simulink model "IEEE_39_IBR_Simplified"  (R2023b)
settings: Solver=FixedStepAuto  StartTime=0  StopTime=20  FixedStep=Ts  MaxStep=1/60  RelTol=1e-3  AbsTol=1e-2  EnableMultiTasking=on
PreLoadFcn:
  | NE39bus_data;
  | PSSMODEL=1;
  | LPSS=0;
  | WAPSS=0;
  | WAPSS2=0;
values from neighbouring files (symbols this model uses):
  Dt = 0    [SG_para.m]
  dw0_sm = 0    [SG_para.m]
  Emax = 1    [SG_para.m]
  Emin = 0.5    [SG_para.m]
  Fg = [0.1,0.1,0.1]    [SG_para.m]
  fn_sm = 60*ones(1,10)    [SG_para.m]
  H_sm = [5,3.03,3.58,2.86,2.6,3.48,2.64,2.43,3.45,4.2]*10    [SG_para.m]
  ia0_sm = 0.75*0    (= 0)    [SG_para.m]
  ib0_sm = 0.75*0    (= 0)    [SG_para.m]
  ic0_sm = 0.75*0    (= 0)    [SG_para.m]
  Kd_sm = 6*ones(1,10)    [SG_para.m]
  Ke = 200    [SG_para.m]
  Kg = [0.95,0.95,0.95]    [SG_para.m]
  Ks = 2    [SG_para.m]
  line = [     1	2	0.0035	0.0411	0.6987	0	100	345 ... (first row only)    [SG_para.m]
  p = 1    [SG_para.m]
  pha0_sm = -24.95*0    (= 0)    [SG_para.m]
  phb0_sm = -144.94*0    (= 0)    [SG_para.m]
  phc0_sm = 95.05*0    (= 0)    [SG_para.m]
  Pn_sm = [1000,1000,1000,1000,1000,1000,1000,1000,1000,1000]    [SG_para.m]
  Pref_sm = [1000 520.81 650 632 508 650 560 540 830 250]./Pn_sm    [SG_para.m]
  R = 1e-3    (= 0.001)    [SG_para.m]
  Rg = [0.05,0.05,0.05]    [SG_para.m]
  rs = 2.8544e-3    (= 0.0028544)    [SG_para.m]
  s = 1    [SG_para.m]
  s1 = 10    [SG_para.m]
  T1 = 0.05    [SG_para.m]
  T2 = 0.5    [SG_para.m]
  T3 = 0.5    [SG_para.m]
  Te = 0.05    [SG_para.m]
  Tfa = 3    [SG_para.m]
  Tfb = 10    [SG_para.m]
  Tg = [10,10,10]    [SG_para.m]
  theta0_sm = -94.3*0    (= 0)    [SG_para.m]
  Ts = 5e-5    (= 5e-05)    [SG_para.m]
  Ts1 = 0.18    [SG_para.m]
  Ts2 = 2    [SG_para.m]
  Ts3 = 5    [SG_para.m]
  Ts4 = 10    [SG_para.m]
  Ts5 = 15    [SG_para.m]
  Un_sm = [345,22,22,22,22,22,22,22,345,22]    [SG_para.m]
  Vmax = inf    [SG_para.m]
  Vmin = 0    [SG_para.m]
  Vref_sm = 1*ones(1,10)    [SG_para.m]
  xd = xd_t    (= 0.296)    [SG_para.m]
undefined symbols (not defined in the file or in its folder): D1, D11, Delta, Ka, Kf, Ta, Tf
libraries: spsThreePhaseVIMeasurementLib x41, spsThreePhaseFaultLib x39, spsThreePhaseSeriesRLCBranchLib x36, spsThreePhaseParallelRLCLoadLib x20, spsThreePhaseTransformerTwoWindingsLib x13, spsSimplifiedSynchronousMachinepuUnitsLib x10, spsLoadFlowBusLib x10, Inverter_based_Resources_IBRs x10, spsThreePhaseBreakerLib x2, spsSequenceAnalyzerLib x2, spsMultimeterLib x1, eePowerMeasurement x1
(part 4 of 5)

== system IEEE_39_IBR_Simplified/A2/G1 ==
  Controllers : Subsystem
  Simplified Synchronous Machine pu Units : spsSimplifiedSynchronousMachinepuUnitsLib/Simplified Synchronous Machine pu Units  ConnectionType=3-wire Y  MechanicalLoad=Mechanical power Pm  MeasurementBus=off  NominalParameters="[ Pn_sm(1)*1e6  Un_sm(1)*1e3  fn_sm(1) ]"  Mechanical=[ H_sm(1) Kd_sm(1) p]  InternalRL="[rs  xd]"  InitialConditions=[dw0_sm theta0_sm ia0_sm ib0_sm ic0_sm pha0_sm phb0_sm phc0_sm]  IterativeDiscreteModel=Trapezoidal non iterative  TsBlock=-1  TsPowergui=0  LoadFlowParameters=[1 0 0 0 0]  Units=0  BusType=swing  Pref=0  Qref=0  Qmin=-inf  Qmax=+inf  PLF=0  QLF=0
      settings: LibrarySourceBlock=|
      | sps_lib/Electrical Machines/Simplified Synchronous
      | Machine pu Units
  A : PMIOPort  Side=Left
  B : PMIOPort  Port=2  Side=Left
  C : PMIOPort  Port=3  Side=Left
  wires:
  Controllers/1(Pm) -> Simplified Synchronous Machine pu Units/1
  Simplified Synchronous Machine pu Units/1 -> Controllers/1(m)
  Controllers/2(Vref) -> Simplified Synchronous Machine pu Units/2
  connections:
  A/RConn1 -- Simplified Synchronous Machine pu Units/RConn1
  B/RConn1 -- Simplified Synchronous Machine pu Units/RConn2
  C/RConn1 -- Simplified Synchronous Machine pu Units/RConn3

== system IEEE_39_IBR_Simplified/A2/G2 ==
  Controllers : Subsystem
  Simplified Synchronous Machine pu Units : spsSimplifiedSynchronousMachinepuUnitsLib/Simplified Synchronous Machine pu Units  ConnectionType=3-wire Y  MechanicalLoad=Mechanical power Pm  MeasurementBus=off  NominalParameters="[ Pn_sm(2)*1e6  Un_sm(2)*1e3  fn_sm(2) ]"  Mechanical=[ H_sm(2) Kd_sm(2) p]  InternalRL="[rs  xd]"  InitialConditions=[dw0_sm theta0_sm ia0_sm ib0_sm ic0_sm pha0_sm phb0_sm phc0_sm]  IterativeDiscreteModel=Trapezoidal non iterative  TsBlock=-1  TsPowergui=0  LoadFlowParameters=[1,0,0,0,0]  Units=0  BusType=PV  Pref=0  Qref=0  Qmin=-inf  Qmax=+inf  PLF=0  QLF=0
      settings: LibrarySourceBlock=|
      | sps_lib/Electrical Machines/Simplified Synchronous
      | Machine pu Units
  A : PMIOPort  Side=Left
  B : PMIOPort  Port=2  Side=Left
  C : PMIOPort  Port=3  Side=Left
  wires:
  Controllers/1(Pm) -> Simplified Synchronous Machine pu Units/1
  Simplified Synchronous Machine pu Units/1 -> Controllers/1(m)
  Controllers/2(Vref) -> Simplified Synchronous Machine pu Units/2
  connections:
  Simplified Synchronous Machine pu Units/RConn2 -- B/RConn1
  Simplified Synchronous Machine pu Units/RConn3 -- C/RConn1
  Simplified Synchronous Machine pu Units/RConn1 -- A/RConn1

== system IEEE_39_IBR_Simplified/A2/G3 ==
  Controllers : Subsystem
  Simplified Synchronous Machine pu Units : spsSimplifiedSynchronousMachinepuUnitsLib/Simplified Synchronous Machine pu Units  ConnectionType=3-wire Y  MechanicalLoad=Mechanical power Pm  MeasurementBus=off  NominalParameters="[ Pn_sm(3)*1e6  Un_sm(3)*1e3  fn_sm(3) ]"  Mechanical=[ H_sm(3) Kd_sm(3) p]  InternalRL="[rs  xd]"  InitialConditions=[dw0_sm theta0_sm ia0_sm ib0_sm ic0_sm pha0_sm phb0_sm phc0_sm]  IterativeDiscreteModel=Trapezoidal non iterative  TsBlock=-1  TsPowergui=0  LoadFlowParameters=[1,0,0,0,0]  Units=0  BusType=PV  Pref=0  Qref=0  Qmin=-inf  Qmax=+inf  PLF=0  QLF=0
      settings: LibrarySourceBlock=|
      | sps_lib/Electrical Machines/Simplified Synchronous
      | Machine pu Units
  A : PMIOPort  Side=Left
  B : PMIOPort  Port=2  Side=Left
  C : PMIOPort  Port=3  Side=Left
  wires:
  Controllers/1(Pm) -> Simplified Synchronous Machine pu Units/1
  Simplified Synchronous Machine pu Units/1 -> Controllers/1(m)
  Controllers/2(Vref) -> Simplified Synchronous Machine pu Units/2
  connections:
  Simplified Synchronous Machine pu Units/RConn2 -- B/RConn1
  Simplified Synchronous Machine pu Units/RConn3 -- C/RConn1
  Simplified Synchronous Machine pu Units/RConn1 -- A/RConn1

== system IEEE_39_IBR_Simplified/A3/G4 ==
  Controllers : Subsystem
  Simplified Synchronous Machine pu Units : spsSimplifiedSynchronousMachinepuUnitsLib/Simplified Synchronous Machine pu Units  ConnectionType=3-wire Y  MechanicalLoad=Mechanical power Pm  MeasurementBus=off  NominalParameters="[ Pn_sm(4)*1e6  Un_sm(4)*1e3  fn_sm(4) ]"  Mechanical=[ H_sm(4) Kd_sm(4) p]  InternalRL="[rs  xd]"  InitialConditions=[dw0_sm theta0_sm ia0_sm ib0_sm ic0_sm pha0_sm phb0_sm phc0_sm]  IterativeDiscreteModel=Trapezoidal non iterative  TsBlock=-1  TsPowergui=0  LoadFlowParameters=[1,0,0,0,0]  Units=0  BusType=PV  Pref=0  Qref=0  Qmin=-inf  Qmax=+inf  PLF=0  QLF=0
      settings: LibrarySourceBlock=|
      | sps_lib/Electrical Machines/Simplified Synchronous
      | Machine pu Units
  A : PMIOPort  Side=Left
  B : PMIOPort  Port=2  Side=Left
  C : PMIOPort  Port=3  Side=Left
  wires:
  Controllers/1(Pm) -> Simplified Synchronous Machine pu Units/1
  Simplified Synchronous Machine pu Units/1 -> Controllers/1(m)
  Controllers/2(Vref) -> Simplified Synchronous Machine pu Units/2
  connections:
  Simplified Synchronous Machine pu Units/RConn2 -- B/RConn1
  Simplified Synchronous Machine pu Units/RConn3 -- C/RConn1
  Simplified Synchronous Machine pu Units/RConn1 -- A/RConn1

== system IEEE_39_IBR_Simplified/A3/G5 ==
  Controllers : Subsystem
  Simplified Synchronous Machine pu Units : spsSimplifiedSynchronousMachinepuUnitsLib/Simplified Synchronous Machine pu Units  ConnectionType=3-wire Y  MechanicalLoad=Mechanical power Pm  MeasurementBus=off  NominalParameters="[ Pn_sm(5)*1e6  Un_sm(5)*1e3  fn_sm(5) ]"  Mechanical=[ H_sm(5) Kd_sm(5) p]  InternalRL="[rs  xd]"  InitialConditions=[dw0_sm theta0_sm ia0_sm ib0_sm ic0_sm pha0_sm phb0_sm phc0_sm]  IterativeDiscreteModel=Trapezoidal non iterative  TsBlock=-1  TsPowergui=0  LoadFlowParameters=[1,0,0,0,0]  Units=0  BusType=PV  Pref=0  Qref=0  Qmin=-inf  Qmax=+inf  PLF=0  QLF=0
      settings: LibrarySourceBlock=|
      | sps_lib/Electrical Machines/Simplified Synchronous
      | Machine pu Units
  A : PMIOPort  Side=Left
  B : PMIOPort  Port=2  Side=Left
  C : PMIOPort  Port=3  Side=Left
  wires:
  Controllers/1(Pm) -> Simplified Synchronous Machine pu Units/1
  Simplified Synchronous Machine pu Units/1 -> Controllers/1(m)
  Controllers/2(Vref) -> Simplified Synchronous Machine pu Units/2
  connections:
  Simplified Synchronous Machine pu Units/RConn2 -- B/RConn1
  Simplified Synchronous Machine pu Units/RConn3 -- C/RConn1
  Simplified Synchronous Machine pu Units/RConn1 -- A/RConn1

== system IEEE_39_IBR_Simplified/A3/G6 ==
  Controllers : Subsystem
  Simplified Synchronous Machine pu Units : spsSimplifiedSynchronousMachinepuUnitsLib/Simplified Synchronous Machine pu Units  ConnectionType=3-wire Y  MechanicalLoad=Mechanical power Pm  MeasurementBus=off  NominalParameters="[ Pn_sm(6)*1e6  Un_sm(6)*1e3  fn_sm(6) ]"  Mechanical=[ H_sm(6) Kd_sm(6) p]  InternalRL="[rs  xd]"  InitialConditions=[dw0_sm theta0_sm ia0_sm ib0_sm ic0_sm pha0_sm phb0_sm phc0_sm]  IterativeDiscreteModel=Trapezoidal non iterative  TsBlock=-1  TsPowergui=0  LoadFlowParameters=[1,0,0,0,0]  Units=0  BusType=PV  Pref=0  Qref=0  Qmin=-inf  Qmax=+inf  PLF=0  QLF=0
      settings: LibrarySourceBlock=|
      | sps_lib/Electrical Machines/Simplified Synchronous
      | Machine pu Units
  A : PMIOPort  Side=Left
  B : PMIOPort  Port=2  Side=Left
  C : PMIOPort  Port=3  Side=Left
  wires:
  Controllers/1(Pm) -> Simplified Synchronous Machine pu Units/1
  Simplified Synchronous Machine pu Units/1 -> Controllers/1(m)
  Controllers/2(Vref) -> Simplified Synchronous Machine pu Units/2
  connections:
  Simplified Synchronous Machine pu Units/RConn2 -- B/RConn1
  Simplified Synchronous Machine pu Units/RConn3 -- C/RConn1
  Simplified Synchronous Machine pu Units/RConn1 -- A/RConn1

== system IEEE_39_IBR_Simplified/A3/G7 ==
  Controllers : Subsystem
  Simplified Synchronous Machine pu Units : spsSimplifiedSynchronousMachinepuUnitsLib/Simplified Synchronous Machine pu Units  ConnectionType=3-wire Y  MechanicalLoad=Mechanical power Pm  MeasurementBus=off  NominalParameters="[ Pn_sm(7)*1e6  Un_sm(7)*1e3  fn_sm(7) ]"  Mechanical=[ H_sm(7) Kd_sm(7) p]  InternalRL="[rs  xd]"  InitialConditions=[dw0_sm theta0_sm ia0_sm ib0_sm ic0_sm pha0_sm phb0_sm phc0_sm]  IterativeDiscreteModel=Trapezoidal non iterative  TsBlock=-1  TsPowergui=0  LoadFlowParameters=[1,0,0,0,0]  Units=0  BusType=PV  Pref=0  Qref=0  Qmin=-inf  Qmax=+inf  PLF=0  QLF=0
      settings: LibrarySourceBlock=|
      | sps_lib/Electrical Machines/Simplified Synchronous
      | Machine pu Units
  A : PMIOPort  Side=Left
  B : PMIOPort  Port=2  Side=Left
  C : PMIOPort  Port=3  Side=Left
  wires:
  Controllers/1(Pm) -> Simplified Synchronous Machine pu Units/1
  Simplified Synchronous Machine pu Units/1 -> Controllers/1(m)
  Controllers/2(Vref) -> Simplified Synchronous Machine pu Units/2
  connections:
  Simplified Synchronous Machine pu Units/RConn2 -- B/RConn1
  Simplified Synchronous Machine pu Units/RConn3 -- C/RConn1
  Simplified Synchronous Machine pu Units/RConn1 -- A/RConn1

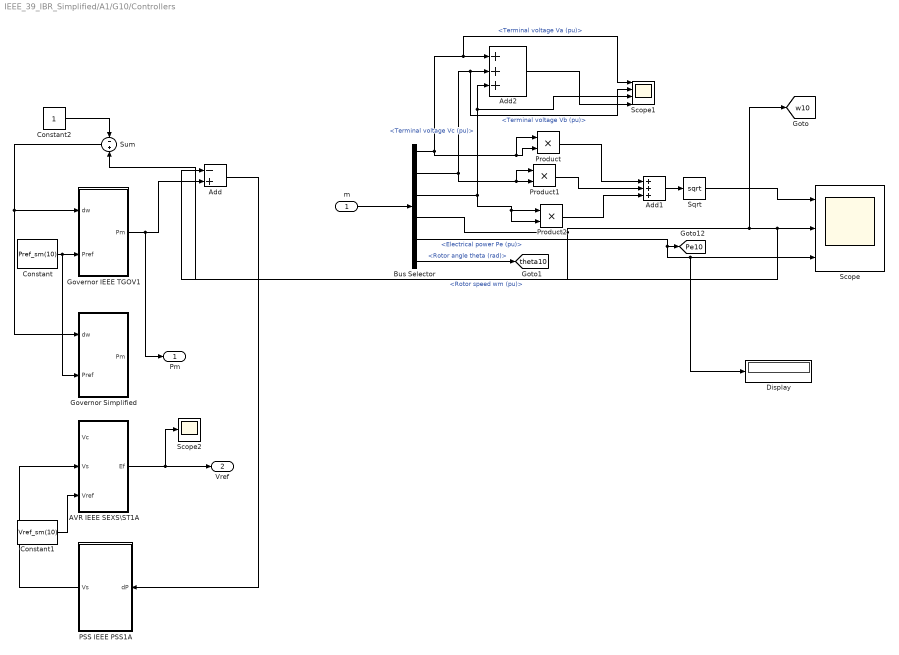
== system IEEE_39_IBR_Simplified/A1/G10/Controllers ==
  m : Inport
  AVR IEEE SEXS\ST1A : Subsystem
  Add : Sum  Inputs=-+
  Add1 : Sum  Inputs=+++
  Add2 : Sum  Inputs=+++
  Bus Selector : BusSelector  OutputSignals=Terminal voltage Va (pu),Terminal voltage Vb (pu),Terminal voltage Vc (pu),Rotor speed wm (pu),Electrical power Pe (pu),Rotor angle theta (rad)
  Constant : Constant  Value=Pref_sm(10)
  Constant1 : Constant  Value=Vref_sm(10)
  Constant2 : Constant
  Display : Display
  Governor Simplified : Subsystem
  Governor IEEE TGOV1 : Subsystem
  PSS IEEE PSS1A : Subsystem
  Product : Product
  Product1 : Product
  Product2 : Product
  Scope : Scope  NumInputPorts=3
  Scope1 : Scope  NumInputPorts=4
  Scope2 : Scope
  Sqrt : Sqrt
  Sum : Sum  Inputs=-+
  Pm : Outport  VectorParamsAs1DForOutWhenUnconnected=off
  Vref : Outport  Port=2  VectorParamsAs1DForOutWhenUnconnected=off
  tag scope: Pe10=global, theta10=global, w10=global
  wires:
  Governor IEEE TGOV1/1(Pm) -> Pm/1, Add/2
  Constant/1 -> Governor Simplified/2(Pref), Governor IEEE TGOV1/2(Pref)
  Add/1 -> PSS IEEE PSS1A/1(dP)
  Constant1/1 -> AVR IEEE SEXS\ST1A/3(Vref)
  PSS IEEE PSS1A/1(Vs) -> AVR IEEE SEXS\ST1A/2(Vs)
  m/1 -> Bus Selector/1
  Bus Selector/4 -> [w10], Sum/2, Scope/2, Add/1  "<Rotor speed wm (pu)>"
  Bus Selector/2 -> Product1/1, Product1/2, Scope1/2, Add2/2  "<Terminal voltage Vb (pu)>"
  Bus Selector/3 -> Product2/1, Product2/2, Scope1/3, Add2/3  "<Terminal voltage Vc (pu)>"
  Bus Selector/1 -> Product/1, Product/2, Scope1/1, Add2/1  "<Terminal voltage Va (pu)>"
  Bus Selector/5 -> Display/1, Scope/3, [Pe10]  "<Electrical power Pe (pu)>"
  Add1/1 -> Sqrt/1
  Product/1 -> Add1/1
  Product1/1 -> Add1/2
  Product2/1 -> Add1/3
  Constant2/1 -> Sum/1
  Sum/1 -> Governor IEEE TGOV1/1(dw), Governor Simplified/1(dw)
  Sqrt/1 -> Scope/1
  Add2/1 -> Scope1/4
  Bus Selector/6 -> [theta10]  "<Rotor angle theta (rad)>"
  AVR IEEE SEXS\ST1A/1(Ef) -> Scope2/1, Vref/1

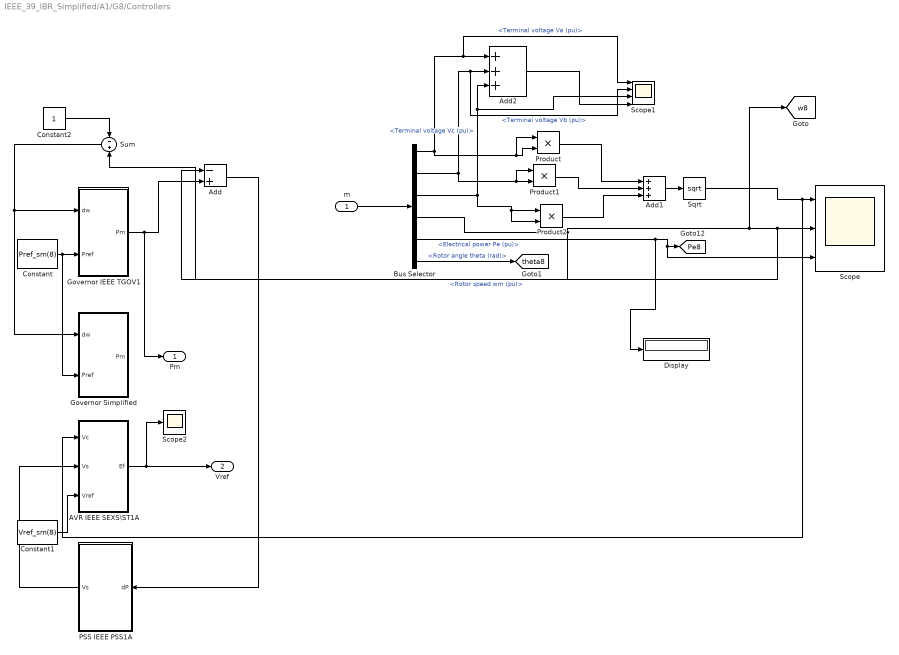
== system IEEE_39_IBR_Simplified/A1/G8/Controllers ==
  m : Inport
  AVR IEEE SEXS\ST1A : Subsystem
  Add : Sum  Inputs=-+
  Add1 : Sum  Inputs=+++
  Add2 : Sum  Inputs=+++
  Bus Selector : BusSelector  OutputSignals=Terminal voltage Va (pu),Terminal voltage Vb (pu),Terminal voltage Vc (pu),Rotor speed wm (pu),Electrical power Pe (pu),Rotor angle theta (rad)
  Constant : Constant  Value=Pref_sm(8)
  Constant1 : Constant  Value=Vref_sm(8)
  Constant2 : Constant
  Display : Display
  Governor Simplified : Subsystem
  Governor IEEE TGOV1 : Subsystem
  PSS IEEE PSS1A : Subsystem
  Product : Product
  Product1 : Product
  Product2 : Product
  Scope : Scope  NumInputPorts=3
  Scope1 : Scope  NumInputPorts=4
  Scope2 : Scope
  Sqrt : Sqrt
  Sum : Sum  Inputs=-+
  Pm : Outport  VectorParamsAs1DForOutWhenUnconnected=off
  Vref : Outport  Port=2  VectorParamsAs1DForOutWhenUnconnected=off
  tag scope: Pe8=global, theta8=global, w8=global
  wires:
  Governor IEEE TGOV1/1(Pm) -> Pm/1, Add/2
  Constant/1 -> Governor Simplified/2(Pref), Governor IEEE TGOV1/2(Pref)
  Add/1 -> PSS IEEE PSS1A/1(dP)
  Constant1/1 -> AVR IEEE SEXS\ST1A/3(Vref)
  PSS IEEE PSS1A/1(Vs) -> AVR IEEE SEXS\ST1A/2(Vs)
  m/1 -> Bus Selector/1
  Bus Selector/4 -> [w8], Sum/2, Scope/2, Add/1  "<Rotor speed wm (pu)>"
  Bus Selector/2 -> Product1/1, Product1/2, Scope1/2, Add2/2  "<Terminal voltage Vb (pu)>"
  Bus Selector/3 -> Product2/1, Product2/2, Scope1/3, Add2/3  "<Terminal voltage Vc (pu)>"
  Bus Selector/1 -> Product/1, Product/2, Scope1/1, Add2/1  "<Terminal voltage Va (pu)>"
  Bus Selector/5 -> Display/1, Scope/3, [Pe8]  "<Electrical power Pe (pu)>"
  Add1/1 -> Sqrt/1
  Product/1 -> Add1/1
  Product1/1 -> Add1/2
  Product2/1 -> Add1/3
  Constant2/1 -> Sum/1
  Sum/1 -> Governor IEEE TGOV1/1(dw), Governor Simplified/1(dw)
  Sqrt/1 -> AVR IEEE SEXS\ST1A/1(Vc), Scope/1
  Add2/1 -> Scope1/4
  Bus Selector/6 -> [theta8]  "<Rotor angle theta (rad)>"
  AVR IEEE SEXS\ST1A/1(Ef) -> Scope2/1, Vref/1

== system IEEE_39_IBR_Simplified/A1/G9/Controllers ==
  m : Inport
  AVR IEEE SEXS\ST1A : Subsystem
  Add : Sum  Inputs=-+
  Add1 : Sum  Inputs=+++
  Add2 : Sum  Inputs=+++
  Bus Selector : BusSelector  OutputSignals=Terminal voltage Va (pu),Terminal voltage Vb (pu),Terminal voltage Vc (pu),Rotor speed wm (pu),Electrical power Pe (pu),Rotor angle theta (rad)
  Constant : Constant  Value=Pref_sm(9)
  Constant1 : Constant  Value=Vref_sm(9)
  Constant2 : Constant
  Display : Display
  Governor Simplified : Subsystem
  Governor IEEE TGOV1 : Subsystem
  PSS IEEE PSS1A : Subsystem
  Product : Product
  Product1 : Product
  Product2 : Product
  Scope : Scope  NumInputPorts=3
  Scope1 : Scope  NumInputPorts=4
  Sqrt : Sqrt
  Sum : Sum  Inputs=-+
  Pm : Outport  VectorParamsAs1DForOutWhenUnconnected=off
  Vref : Outport  Port=2  VectorParamsAs1DForOutWhenUnconnected=off
  tag scope: Pe9=global, theta9=global, w9=global
  wires:
  Governor IEEE TGOV1/1(Pm) -> Pm/1, Add/2
  Constant/1 -> Governor Simplified/2(Pref), Governor IEEE TGOV1/2(Pref)
  Add/1 -> PSS IEEE PSS1A/1(dP)
  Constant1/1 -> AVR IEEE SEXS\ST1A/3(Vref)
  PSS IEEE PSS1A/1(Vs) -> AVR IEEE SEXS\ST1A/2(Vs)
  m/1 -> Bus Selector/1
  Bus Selector/4 -> [w9], Sum/2, Scope/2, Add/1  "<Rotor speed wm (pu)>"
  Bus Selector/2 -> Product1/1, Product1/2, Scope1/2, Add2/2  "<Terminal voltage Vb (pu)>"
  Bus Selector/3 -> Product2/1, Product2/2, Scope1/3, Add2/3  "<Terminal voltage Vc (pu)>"
  Bus Selector/1 -> Product/1, Product/2, Scope1/1, Add2/1  "<Terminal voltage Va (pu)>"
  Bus Selector/5 -> Display/1, Scope/3, [Pe9]  "<Electrical power Pe (pu)>"
  Add1/1 -> Sqrt/1
  Product/1 -> Add1/1
  Product1/1 -> Add1/2
  Product2/1 -> Add1/3
  Constant2/1 -> Sum/1
  Sum/1 -> Governor IEEE TGOV1/1(dw), Governor Simplified/1(dw)
  Sqrt/1 -> Scope/1
  Add2/1 -> Scope1/4
  Bus Selector/6 -> [theta9]  "<Rotor angle theta (rad)>"
  AVR IEEE SEXS\ST1A/1(Ef) -> Vref/1

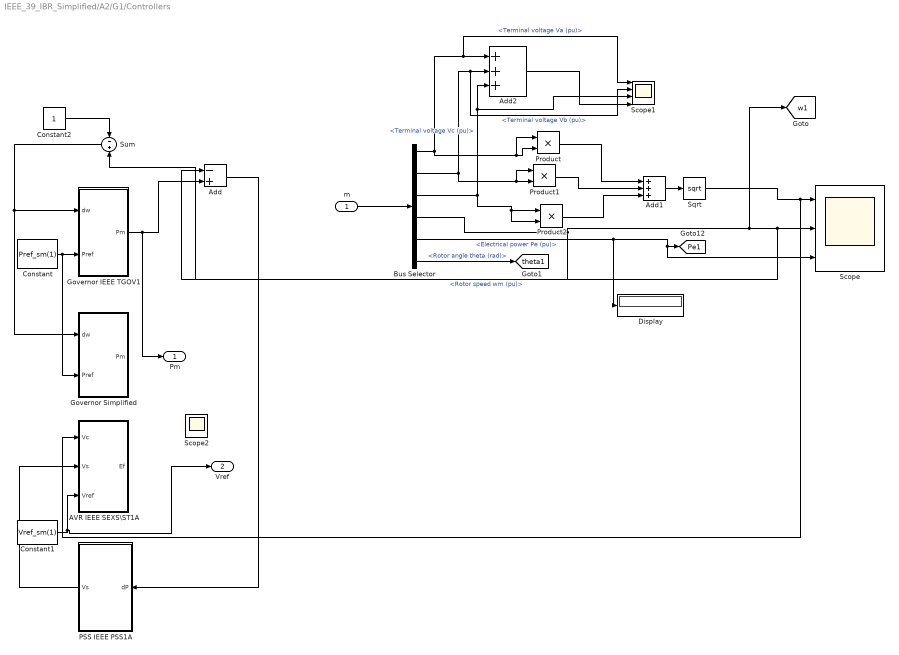
== system IEEE_39_IBR_Simplified/A2/G1/Controllers ==
  m : Inport
  AVR IEEE SEXS\ST1A : Subsystem
  Add : Sum  Inputs=-+
  Add1 : Sum  Inputs=+++
  Add2 : Sum  Inputs=+++
  Bus Selector : BusSelector  OutputSignals=Terminal voltage Va (pu),Terminal voltage Vb (pu),Terminal voltage Vc (pu),Rotor speed wm (pu),Electrical power Pe (pu),Rotor angle theta (rad)
  Constant : Constant  Value=Pref_sm(1)
  Constant1 : Constant  Value=Vref_sm(1)
  Constant2 : Constant
  Display : Display
  Governor Simplified : Subsystem
  Governor IEEE TGOV1 : Subsystem
  PSS IEEE PSS1A : Subsystem
  Product : Product
  Product1 : Product
  Product2 : Product
  Scope : Scope  NumInputPorts=3
  Scope1 : Scope  NumInputPorts=4
  Scope2 : Scope
  Sqrt : Sqrt
  Sum : Sum  Inputs=-+
  Pm : Outport  VectorParamsAs1DForOutWhenUnconnected=off
  Vref : Outport  Port=2  VectorParamsAs1DForOutWhenUnconnected=off
  tag scope: Pe1=global, theta1=global, w1=global
  wires:
  Governor IEEE TGOV1/1(Pm) -> Pm/1, Add/2
  Constant/1 -> Governor Simplified/2(Pref), Governor IEEE TGOV1/2(Pref)
  Add/1 -> PSS IEEE PSS1A/1(dP)
  Constant1/1 -> Vref/1, AVR IEEE SEXS\ST1A/3(Vref)
  PSS IEEE PSS1A/1(Vs) -> AVR IEEE SEXS\ST1A/2(Vs)
  m/1 -> Bus Selector/1
  Bus Selector/4 -> [w1], Sum/2, Scope/2, Add/1  "<Rotor speed wm (pu)>"
  Bus Selector/2 -> Product1/1, Product1/2, Scope1/2, Add2/2  "<Terminal voltage Vb (pu)>"
  Bus Selector/3 -> Product2/1, Product2/2, Scope1/3, Add2/3  "<Terminal voltage Vc (pu)>"
  Bus Selector/1 -> Product/1, Product/2, Scope1/1, Add2/1  "<Terminal voltage Va (pu)>"
  Bus Selector/5 -> Display/1, Scope/3, [Pe1]  "<Electrical power Pe (pu)>"
  Add1/1 -> Sqrt/1
  Product/1 -> Add1/1
  Product1/1 -> Add1/2
  Product2/1 -> Add1/3
  Constant2/1 -> Sum/1
  Sum/1 -> Governor IEEE TGOV1/1(dw), Governor Simplified/1(dw)
  Sqrt/1 -> AVR IEEE SEXS\ST1A/1(Vc), Scope/1
  Add2/1 -> Scope1/4
  Bus Selector/6 -> [theta1]  "<Rotor angle theta (rad)>"

== system IEEE_39_IBR_Simplified/A2/G2/Controllers ==
  m : Inport
  AVR IEEE SEXS\ST1A : Subsystem
  Add : Sum  Inputs=-+
  Add1 : Sum  Inputs=+++
  Add2 : Sum  Inputs=+++
  Bus Selector : BusSelector  OutputSignals=Terminal voltage Va (pu),Terminal voltage Vb (pu),Terminal voltage Vc (pu),Rotor speed wm (pu),Electrical power Pe (pu),Rotor angle theta (rad)
  Constant : Constant  Value=Pref_sm(2)
  Constant1 : Constant  Value=Vref_sm(2)
  Constant2 : Constant
  Display : Display
  Governor Simplified : Subsystem
  Governor IEEE TGOV1 : Subsystem
  PSS IEEE PSS1A : Subsystem
  Product : Product
  Product1 : Product
  Product2 : Product
  Scope : Scope  NumInputPorts=3
  Scope1 : Scope  NumInputPorts=4
  Sqrt : Sqrt
  Sum : Sum  Inputs=-+
  Pm : Outport  VectorParamsAs1DForOutWhenUnconnected=off
  Vref : Outport  Port=2  VectorParamsAs1DForOutWhenUnconnected=off
  tag scope: Pe2=global, theta2=global, w2=global
  wires:
  Governor IEEE TGOV1/1(Pm) -> Pm/1, Add/2
  Constant/1 -> Governor Simplified/2(Pref), Governor IEEE TGOV1/2(Pref)
  Add/1 -> PSS IEEE PSS1A/1(dP)
  Constant1/1 -> AVR IEEE SEXS\ST1A/3(Vref)
  PSS IEEE PSS1A/1(Vs) -> AVR IEEE SEXS\ST1A/2(Vs)
  m/1 -> Bus Selector/1
  Bus Selector/4 -> [w2], Sum/2, Scope/2, Add/1  "<Rotor speed wm (pu)>"
  Bus Selector/2 -> Product1/1, Product1/2, Scope1/2, Add2/2  "<Terminal voltage Vb (pu)>"
  Bus Selector/3 -> Product2/1, Product2/2, Scope1/3, Add2/3  "<Terminal voltage Vc (pu)>"
  Bus Selector/1 -> Product/1, Product/2, Scope1/1, Add2/1  "<Terminal voltage Va (pu)>"
  Bus Selector/5 -> Display/1, Scope/3, [Pe2]  "<Electrical power Pe (pu)>"
  Add1/1 -> Sqrt/1
  Product/1 -> Add1/1
  Product1/1 -> Add1/2
  Product2/1 -> Add1/3
  Constant2/1 -> Sum/1
  Sum/1 -> Governor IEEE TGOV1/1(dw), Governor Simplified/1(dw)
  Sqrt/1 -> Scope/1
  Add2/1 -> Scope1/4
  Bus Selector/6 -> [theta2]  "<Rotor angle theta (rad)>"
  AVR IEEE SEXS\ST1A/1(Ef) -> Vref/1

== system IEEE_39_IBR_Simplified/A2/G3/Controllers ==
  m : Inport
  AVR IEEE SEXS\ST1A : Subsystem
  Add : Sum  Inputs=-+
  Add1 : Sum  Inputs=+++
  Add2 : Sum  Inputs=+++
  Bus Selector : BusSelector  OutputSignals=Terminal voltage Va (pu),Terminal voltage Vb (pu),Terminal voltage Vc (pu),Rotor speed wm (pu),Electrical power Pe (pu),Rotor angle theta (rad)
  Constant : Constant  Value=Pref_sm(3)
  Constant1 : Constant  Value=Vref_sm(3)
  Constant2 : Constant
  Display : Display
  Governor Simplified : Subsystem
  Governor IEEE TGOV1 : Subsystem
  PSS IEEE PSS1A : Subsystem
  Product : Product
  Product1 : Product
  Product2 : Product
  Scope : Scope  NumInputPorts=3
  Scope1 : Scope  NumInputPorts=4
  Sqrt : Sqrt
  Sum : Sum  Inputs=-+
  Pm : Outport  VectorParamsAs1DForOutWhenUnconnected=off
  Vref : Outport  Port=2  VectorParamsAs1DForOutWhenUnconnected=off
  tag scope: Pe3=global, theta3=global, w3=global
  wires:
  Governor IEEE TGOV1/1(Pm) -> Pm/1, Add/2
  Constant/1 -> Governor Simplified/2(Pref), Governor IEEE TGOV1/2(Pref)
  Add/1 -> PSS IEEE PSS1A/1(dP)
  Constant1/1 -> AVR IEEE SEXS\ST1A/3(Vref)
  PSS IEEE PSS1A/1(Vs) -> AVR IEEE SEXS\ST1A/2(Vs)
  m/1 -> Bus Selector/1
  Bus Selector/4 -> [w3], Sum/2, Scope/2, Add/1  "<Rotor speed wm (pu)>"
  Bus Selector/2 -> Product1/1, Product1/2, Scope1/2, Add2/2  "<Terminal voltage Vb (pu)>"
  Bus Selector/3 -> Product2/1, Product2/2, Scope1/3, Add2/3  "<Terminal voltage Vc (pu)>"
  Bus Selector/1 -> Product/1, Product/2, Scope1/1, Add2/1  "<Terminal voltage Va (pu)>"
  Bus Selector/5 -> Display/1, Scope/3, [Pe3]  "<Electrical power Pe (pu)>"
  Add1/1 -> Sqrt/1
  Product/1 -> Add1/1
  Product1/1 -> Add1/2
  Product2/1 -> Add1/3
  Constant2/1 -> Sum/1
  Sum/1 -> Governor IEEE TGOV1/1(dw), Governor Simplified/1(dw)
  Sqrt/1 -> Scope/1
  Add2/1 -> Scope1/4
  Bus Selector/6 -> [theta3]  "<Rotor angle theta (rad)>"
  AVR IEEE SEXS\ST1A/1(Ef) -> Vref/1

== system IEEE_39_IBR_Simplified/A3/G4/Controllers ==
  m : Inport
  AVR IEEE SEXS\ST1A : Subsystem
  Add : Sum  Inputs=-+
  Add1 : Sum  Inputs=+++
  Add2 : Sum  Inputs=+++
  Bus Selector : BusSelector  OutputSignals=Terminal voltage Va (pu),Terminal voltage Vb (pu),Terminal voltage Vc (pu),Rotor speed wm (pu),Electrical power Pe (pu),Rotor angle theta (rad)
  Constant : Constant  Value=Pref_sm(4)
  Constant1 : Constant  Value=Vref_sm(4)
  Constant2 : Constant
  Display : Display
  Governor Simplified : Subsystem
  Governor IEEE TGOV1 : Subsystem
  PSS IEEE PSS1A : Subsystem
  Product : Product
  Product1 : Product
  Product2 : Product
  Scope : Scope  NumInputPorts=3
  Scope1 : Scope  NumInputPorts=4
  Sqrt : Sqrt
  Sum : Sum  Inputs=-+
  Pm : Outport  VectorParamsAs1DForOutWhenUnconnected=off
  Vref : Outport  Port=2  VectorParamsAs1DForOutWhenUnconnected=off
  tag scope: Pe4=global, theta4=global, w4=global
  wires:
  Governor IEEE TGOV1/1(Pm) -> Pm/1, Add/2
  Constant/1 -> Governor Simplified/2(Pref), Governor IEEE TGOV1/2(Pref)
  Add/1 -> PSS IEEE PSS1A/1(dP)
  Constant1/1 -> AVR IEEE SEXS\ST1A/3(Vref)
  PSS IEEE PSS1A/1(Vs) -> AVR IEEE SEXS\ST1A/2(Vs)
  m/1 -> Bus Selector/1
  Bus Selector/4 -> [w4], Sum/2, Scope/2, Add/1  "<Rotor speed wm (pu)>"
  Bus Selector/2 -> Product1/1, Product1/2, Scope1/2, Add2/2  "<Terminal voltage Vb (pu)>"
  Bus Selector/3 -> Product2/1, Product2/2, Scope1/3, Add2/3  "<Terminal voltage Vc (pu)>"
  Bus Selector/1 -> Product/1, Product/2, Scope1/1, Add2/1  "<Terminal voltage Va (pu)>"
  Bus Selector/5 -> Display/1, Scope/3, [Pe4]  "<Electrical power Pe (pu)>"
  Add1/1 -> Sqrt/1
  Product/1 -> Add1/1
  Product1/1 -> Add1/2
  Product2/1 -> Add1/3
  Constant2/1 -> Sum/1
  Sum/1 -> Governor IEEE TGOV1/1(dw), Governor Simplified/1(dw)
  Sqrt/1 -> Scope/1
  Add2/1 -> Scope1/4
  Bus Selector/6 -> [theta4]  "<Rotor angle theta (rad)>"
  AVR IEEE SEXS\ST1A/1(Ef) -> Vref/1

== system IEEE_39_IBR_Simplified/A3/G5/Controllers ==
  m : Inport
  AVR IEEE SEXS\ST1A : Subsystem
  Add : Sum  Inputs=-+
  Add1 : Sum  Inputs=+++
  Add2 : Sum  Inputs=+++
  Bus Selector : BusSelector  OutputSignals=Terminal voltage Va (pu),Terminal voltage Vb (pu),Terminal voltage Vc (pu),Rotor speed wm (pu),Electrical power Pe (pu),Rotor angle theta (rad)
  Constant : Constant  Value=Pref_sm(5)
  Constant1 : Constant  Value=Vref_sm(5)
  Constant2 : Constant
  Display : Display
  Governor Simplified : Subsystem
  Governor IEEE TGOV1 : Subsystem
  PSS IEEE PSS1A : Subsystem
  Product : Product
  Product1 : Product
  Product2 : Product
  Scope : Scope  NumInputPorts=3
  Scope1 : Scope  NumInputPorts=4
  Sqrt : Sqrt
  Sum : Sum  Inputs=-+
  Pm : Outport  VectorParamsAs1DForOutWhenUnconnected=off
  Vref : Outport  Port=2  VectorParamsAs1DForOutWhenUnconnected=off
  tag scope: Pe5=global, theta5=global, w5=global
  wires:
  Governor IEEE TGOV1/1(Pm) -> Pm/1, Add/2
  Constant/1 -> Governor Simplified/2(Pref), Governor IEEE TGOV1/2(Pref)
  Add/1 -> PSS IEEE PSS1A/1(dP)
  Constant1/1 -> AVR IEEE SEXS\ST1A/3(Vref)
  PSS IEEE PSS1A/1(Vs) -> AVR IEEE SEXS\ST1A/2(Vs)
  m/1 -> Bus Selector/1
  Bus Selector/4 -> [w5], Sum/2, Scope/2, Add/1  "<Rotor speed wm (pu)>"
  Bus Selector/2 -> Product1/1, Product1/2, Scope1/2, Add2/2  "<Terminal voltage Vb (pu)>"
  Bus Selector/3 -> Product2/1, Product2/2, Scope1/3, Add2/3  "<Terminal voltage Vc (pu)>"
  Bus Selector/1 -> Product/1, Product/2, Scope1/1, Add2/1  "<Terminal voltage Va (pu)>"
  Bus Selector/5 -> Display/1, Scope/3, [Pe5]  "<Electrical power Pe (pu)>"
  Add1/1 -> Sqrt/1
  Product/1 -> Add1/1
  Product1/1 -> Add1/2
  Product2/1 -> Add1/3
  Constant2/1 -> Sum/1
  Sum/1 -> Governor IEEE TGOV1/1(dw), Governor Simplified/1(dw)
  Sqrt/1 -> Scope/1
  Add2/1 -> Scope1/4
  Bus Selector/6 -> [theta5]  "<Rotor angle theta (rad)>"
  AVR IEEE SEXS\ST1A/1(Ef) -> Vref/1

== system IEEE_39_IBR_Simplified/A3/G6/Controllers ==
  m : Inport
  AVR IEEE SEXS\ST1A : Subsystem
  Add : Sum  Inputs=-+
  Add1 : Sum  Inputs=+++
  Add2 : Sum  Inputs=+++
  Bus Selector : BusSelector  OutputSignals=Terminal voltage Va (pu),Terminal voltage Vb (pu),Terminal voltage Vc (pu),Rotor speed wm (pu),Electrical power Pe (pu),Rotor angle theta (rad)
  Constant : Constant  Value=Pref_sm(6)
  Constant1 : Constant  Value=Vref_sm(6)
  Constant2 : Constant
  Display : Display
  Governor Simplified : Subsystem
  Governor IEEE TGOV1 : Subsystem
  PSS IEEE PSS1A : Subsystem
  Product : Product
  Product1 : Product
  Product2 : Product
  Scope : Scope  NumInputPorts=3
  Scope1 : Scope  NumInputPorts=4
  Sqrt : Sqrt
  Sum : Sum  Inputs=-+
  Pm : Outport  VectorParamsAs1DForOutWhenUnconnected=off
  Vref : Outport  Port=2  VectorParamsAs1DForOutWhenUnconnected=off
  tag scope: Pe6=global, theta6=global, w6=global
  wires:
  Governor IEEE TGOV1/1(Pm) -> Pm/1, Add/2
  Constant/1 -> Governor Simplified/2(Pref), Governor IEEE TGOV1/2(Pref)
  Add/1 -> PSS IEEE PSS1A/1(dP)
  Constant1/1 -> AVR IEEE SEXS\ST1A/3(Vref)
  PSS IEEE PSS1A/1(Vs) -> AVR IEEE SEXS\ST1A/2(Vs)
  m/1 -> Bus Selector/1
  Bus Selector/4 -> [w6], Sum/2, Scope/2, Add/1  "<Rotor speed wm (pu)>"
  Bus Selector/2 -> Product1/1, Product1/2, Scope1/2, Add2/2  "<Terminal voltage Vb (pu)>"
  Bus Selector/3 -> Product2/1, Product2/2, Scope1/3, Add2/3  "<Terminal voltage Vc (pu)>"
  Bus Selector/1 -> Product/1, Product/2, Scope1/1, Add2/1  "<Terminal voltage Va (pu)>"
  Bus Selector/5 -> Display/1, Scope/3, [Pe6]  "<Electrical power Pe (pu)>"
  Add1/1 -> Sqrt/1
  Product/1 -> Add1/1
  Product1/1 -> Add1/2
  Product2/1 -> Add1/3
  Constant2/1 -> Sum/1
  Sum/1 -> Governor IEEE TGOV1/1(dw), Governor Simplified/1(dw)
  Sqrt/1 -> Scope/1
  Add2/1 -> Scope1/4
  Bus Selector/6 -> [theta6]  "<Rotor angle theta (rad)>"
  AVR IEEE SEXS\ST1A/1(Ef) -> Vref/1

== system IEEE_39_IBR_Simplified/A3/G7/Controllers ==
  m : Inport
  AVR IEEE SEXS\ST1A : Subsystem
  Add : Sum  Inputs=-+
  Add1 : Sum  Inputs=+++
  Add2 : Sum  Inputs=+++
  Bus Selector : BusSelector  OutputSignals=Terminal voltage Va (pu),Terminal voltage Vb (pu),Terminal voltage Vc (pu),Rotor speed wm (pu),Electrical power Pe (pu),Rotor angle theta (rad)
  Constant : Constant  Value=Pref_sm(7)
  Constant1 : Constant  Value=Vref_sm(7)
  Constant2 : Constant
  Display : Display
  Governor Simplified : Subsystem
  Governor IEEE TGOV1 : Subsystem
  PSS IEEE PSS1A : Subsystem
  Product : Product
  Product1 : Product
  Product2 : Product
  Scope : Scope  NumInputPorts=3
  Scope1 : Scope  NumInputPorts=4
  Sqrt : Sqrt
  Sum : Sum  Inputs=-+
  Pm : Outport  VectorParamsAs1DForOutWhenUnconnected=off
  Vref : Outport  Port=2  VectorParamsAs1DForOutWhenUnconnected=off
  tag scope: Pe7=global, theta7=global, w7=global
  wires:
  Governor IEEE TGOV1/1(Pm) -> Pm/1, Add/2
  Constant/1 -> Governor Simplified/2(Pref), Governor IEEE TGOV1/2(Pref)
  Add/1 -> PSS IEEE PSS1A/1(dP)
  Constant1/1 -> AVR IEEE SEXS\ST1A/3(Vref)
  PSS IEEE PSS1A/1(Vs) -> AVR IEEE SEXS\ST1A/2(Vs)
  m/1 -> Bus Selector/1
  Bus Selector/4 -> [w7], Sum/2, Scope/2, Add/1  "<Rotor speed wm (pu)>"
  Bus Selector/2 -> Product1/1, Product1/2, Scope1/2, Add2/2  "<Terminal voltage Vb (pu)>"
  Bus Selector/3 -> Product2/1, Product2/2, Scope1/3, Add2/3  "<Terminal voltage Vc (pu)>"
  Bus Selector/1 -> Product/1, Product/2, Scope1/1, Add2/1  "<Terminal voltage Va (pu)>"
  Bus Selector/5 -> Display/1, Scope/3, [Pe7]  "<Electrical power Pe (pu)>"
  Add1/1 -> Sqrt/1
  Product/1 -> Add1/1
  Product1/1 -> Add1/2
  Product2/1 -> Add1/3
  Constant2/1 -> Sum/1
  Sum/1 -> Governor IEEE TGOV1/1(dw), Governor Simplified/1(dw)
  Sqrt/1 -> Scope/1
  Add2/1 -> Scope1/4
  Bus Selector/6 -> [theta7]  "<Rotor angle theta (rad)>"
  AVR IEEE SEXS\ST1A/1(Ef) -> Vref/1

== system IEEE_39_IBR_Simplified/A1/G10/Controllers/AVR IEEE SEXS\ST1A ==
  Vc : Inport
  Vs : Inport  Port=2
  Vref : Inport  Port=3
  AVR IEEE ST1a : Subsystem  Commented=on
  AVR SEXS : Subsystem
  Sum1 : Sum  Inputs=+-+
  Ef : Outport  VectorParamsAs1DForOutWhenUnconnected=off
  wires:
  Vc/1 -> Sum1/2
  Vref/1 -> Sum1/1
  Vs/1 -> Sum1/3
  Sum1/1 -> AVR SEXS/1(dV)
  AVR SEXS/1(Ef) -> Ef/1

== system IEEE_39_IBR_Simplified/A1/G10/Controllers/Governor Simplified ==
  dw : Inport
  Pref : Inport  Port=2
  Gain : Gain  Gain=Kg(1)/Rg(1)
  Saturation : Saturate  UpperLimit=Vmax  LowerLimit=Vmin
  Sum1 : Sum  Inputs=|+-
  Transfer Fcn : TransferFcn  Numerator=[Fg(1)*Tg(1) 1]  Denominator=[Tg(1) 1]
  Pm : Outport  VectorParamsAs1DForOutWhenUnconnected=off
  wires:
  Transfer Fcn/1 -> Gain/1
  dw/1 -> Transfer Fcn/1
  Pref/1 -> Sum1/1
  Sum1/1 -> Saturation/1
  Gain/1 -> Sum1/2
  Saturation/1 -> Pm/1

== system IEEE_39_IBR_Simplified/A1/G10/Controllers/Governor IEEE TGOV1 ==
  dw : Inport
  Pref : Inport  Port=2
  Gain : Gain  Gain=1/R
  Gain1 : Gain  Gain=Dt
  Saturation : Saturate  UpperLimit=Vmax  LowerLimit=Vmin
  Scope : Scope  NumInputPorts=3
  Sum : Sum  Inputs=|+-
  Sum1 : Sum  Inputs=|+-
  Transfer Fcn : TransferFcn  Denominator=[T1 1]
  Transfer Fcn1 : TransferFcn  Numerator=[T2 1]  Denominator=[T3 1]
  Pm : Outport  VectorParamsAs1DForOutWhenUnconnected=off
  wires:
  Transfer Fcn/1 -> Saturation/1
  Sum1/1 -> Scope/2, Transfer Fcn/1
  Gain1/1 -> Sum/2
  Saturation/1 -> Transfer Fcn1/1
  Sum/1 -> Pm/1
  dw/1 -> Gain1/1, Gain/1
  Transfer Fcn1/1 -> Scope/3, Sum/1
  Gain/1 -> Sum1/2
  Pref/1 -> Scope/1, Sum1/1

== system IEEE_39_IBR_Simplified/A1/G10/Controllers/PSS IEEE PSS1A ==
  dP : Inport
  Gain : Gain  Gain=Ks
  Transfer Fcn : TransferFcn  Numerator=[Ts1 1]  Denominator=[Ts2 1]
  Transfer Fcn1 : TransferFcn  Numerator=[Ts5 0]  Denominator=[Ts5 1]
  Transfer Fcn2 : TransferFcn  Numerator=[Ts3 1]  Denominator=[Ts4 1]
  Vs : Outport  VectorParamsAs1DForOutWhenUnconnected=off
  wires:
  Transfer Fcn/1 -> Transfer Fcn2/1
  Gain/1 -> Transfer Fcn1/1
  dP/1 -> Transfer Fcn/1
  Transfer Fcn2/1 -> Gain/1
  Transfer Fcn1/1 -> Vs/1

== system IEEE_39_IBR_Simplified/A1/G8/Controllers/AVR IEEE SEXS\ST1A ==
  Vc : Inport
  Vs : Inport  Port=2
  Vref : Inport  Port=3
  AVR IEEE ST1a : Subsystem  Commented=on
  AVR SEXS : Subsystem
  Sum1 : Sum  Inputs=+-+
  Ef : Outport  VectorParamsAs1DForOutWhenUnconnected=off
  wires:
  Vc/1 -> Sum1/2
  Vref/1 -> Sum1/1
  Vs/1 -> Sum1/3
  Sum1/1 -> AVR SEXS/1(dV)
  AVR SEXS/1(Ef) -> Ef/1

== system IEEE_39_IBR_Simplified/A1/G8/Controllers/Governor Simplified ==
  dw : Inport
  Pref : Inport  Port=2
  Gain : Gain  Gain=Kg(1)/Rg(1)
  Saturation : Saturate  UpperLimit=Vmax  LowerLimit=Vmin
  Sum1 : Sum  Inputs=|+-
  Transfer Fcn : TransferFcn  Numerator=[Fg(1)*Tg(1) 1]  Denominator=[Tg(1) 1]
  Pm : Outport  VectorParamsAs1DForOutWhenUnconnected=off
  wires:
  Transfer Fcn/1 -> Gain/1
  dw/1 -> Transfer Fcn/1
  Pref/1 -> Sum1/1
  Sum1/1 -> Saturation/1
  Gain/1 -> Sum1/2
  Saturation/1 -> Pm/1

== system IEEE_39_IBR_Simplified/A1/G8/Controllers/Governor IEEE TGOV1 ==
  dw : Inport
  Pref : Inport  Port=2
  Gain : Gain  Gain=1/R
  Gain1 : Gain  Gain=Dt
  Saturation : Saturate  UpperLimit=Vmax  LowerLimit=Vmin
  Scope : Scope  NumInputPorts=3
  Sum : Sum  Inputs=|+-
  Sum1 : Sum  Inputs=|+-
  Transfer Fcn : TransferFcn  Denominator=[T1 1]
  Transfer Fcn1 : TransferFcn  Numerator=[T2 1]  Denominator=[T3 1]
  Pm : Outport  VectorParamsAs1DForOutWhenUnconnected=off
  wires:
  Transfer Fcn/1 -> Saturation/1
  Sum1/1 -> Scope/2, Transfer Fcn/1
  Gain1/1 -> Sum/2
  Saturation/1 -> Transfer Fcn1/1
  Sum/1 -> Pm/1
  dw/1 -> Gain1/1, Gain/1
  Transfer Fcn1/1 -> Scope/3, Sum/1
  Gain/1 -> Sum1/2
  Pref/1 -> Scope/1, Sum1/1

== system IEEE_39_IBR_Simplified/A1/G8/Controllers/PSS IEEE PSS1A ==
  dP : Inport
  Gain : Gain  Gain=Ks
  Transfer Fcn : TransferFcn  Numerator=[Ts1 1]  Denominator=[Ts2 1]
  Transfer Fcn1 : TransferFcn  Numerator=[Ts5 0]  Denominator=[Ts5 1]
  Transfer Fcn2 : TransferFcn  Numerator=[Ts3 1]  Denominator=[Ts4 1]
  Vs : Outport  VectorParamsAs1DForOutWhenUnconnected=off
  wires:
  Transfer Fcn/1 -> Transfer Fcn2/1
  Gain/1 -> Transfer Fcn1/1
  dP/1 -> Transfer Fcn/1
  Transfer Fcn2/1 -> Gain/1
  Transfer Fcn1/1 -> Vs/1

== system IEEE_39_IBR_Simplified/A1/G9/Controllers/AVR IEEE SEXS\ST1A ==
  Vc : Inport
  Vs : Inport  Port=2
  Vref : Inport  Port=3
  AVR IEEE ST1a : Subsystem  Commented=on
  AVR SEXS : Subsystem
  Sum1 : Sum  Inputs=+-+
  Ef : Outport  VectorParamsAs1DForOutWhenUnconnected=off
  wires:
  Vc/1 -> Sum1/2
  Vref/1 -> Sum1/1
  Vs/1 -> Sum1/3
  Sum1/1 -> AVR SEXS/1(dV)
  AVR SEXS/1(Ef) -> Ef/1

== system IEEE_39_IBR_Simplified/A1/G9/Controllers/Governor Simplified ==
  dw : Inport
  Pref : Inport  Port=2
  Gain : Gain  Gain=Kg(1)/Rg(1)
  Saturation : Saturate  UpperLimit=Vmax  LowerLimit=Vmin
  Sum1 : Sum  Inputs=|+-
  Transfer Fcn : TransferFcn  Numerator=[Fg(1)*Tg(1) 1]  Denominator=[Tg(1) 1]
  Pm : Outport  VectorParamsAs1DForOutWhenUnconnected=off
  wires:
  Transfer Fcn/1 -> Gain/1
  dw/1 -> Transfer Fcn/1
  Pref/1 -> Sum1/1
  Sum1/1 -> Saturation/1
  Gain/1 -> Sum1/2
  Saturation/1 -> Pm/1

== system IEEE_39_IBR_Simplified/A1/G9/Controllers/Governor IEEE TGOV1 ==
  dw : Inport
  Pref : Inport  Port=2
  Gain : Gain  Gain=1/R
  Gain1 : Gain  Gain=Dt
  Saturation : Saturate  UpperLimit=Vmax  LowerLimit=Vmin
  Scope : Scope  NumInputPorts=3
  Sum : Sum  Inputs=|+-
  Sum1 : Sum  Inputs=|+-
  Transfer Fcn : TransferFcn  Denominator=[T1 1]
  Transfer Fcn1 : TransferFcn  Numerator=[T2 1]  Denominator=[T3 1]
  Pm : Outport  VectorParamsAs1DForOutWhenUnconnected=off
  wires:
  Transfer Fcn/1 -> Saturation/1
  Sum1/1 -> Scope/2, Transfer Fcn/1
  Gain1/1 -> Sum/2
  Saturation/1 -> Transfer Fcn1/1
  Sum/1 -> Pm/1
  dw/1 -> Gain1/1, Gain/1
  Transfer Fcn1/1 -> Scope/3, Sum/1
  Gain/1 -> Sum1/2
  Pref/1 -> Scope/1, Sum1/1

== system IEEE_39_IBR_Simplified/A1/G9/Controllers/PSS IEEE PSS1A ==
  dP : Inport
  Gain : Gain  Gain=Ks
  Transfer Fcn : TransferFcn  Numerator=[Ts1 1]  Denominator=[Ts2 1]
  Transfer Fcn1 : TransferFcn  Numerator=[Ts5 0]  Denominator=[Ts5 1]
  Transfer Fcn2 : TransferFcn  Numerator=[Ts3 1]  Denominator=[Ts4 1]
  Vs : Outport  VectorParamsAs1DForOutWhenUnconnected=off
  wires:
  Transfer Fcn/1 -> Transfer Fcn2/1
  Gain/1 -> Transfer Fcn1/1
  dP/1 -> Transfer Fcn/1
  Transfer Fcn2/1 -> Gain/1
  Transfer Fcn1/1 -> Vs/1

== system IEEE_39_IBR_Simplified/A2/G1/Controllers/AVR IEEE SEXS\ST1A ==
  Vc : Inport
  Vs : Inport  Port=2
  Vref : Inport  Port=3
  AVR IEEE ST1a : Subsystem  Commented=on
  AVR SEXS : Subsystem
  Sum1 : Sum  Inputs=+-+
  Ef : Outport  VectorParamsAs1DForOutWhenUnconnected=off
  wires:
  Vc/1 -> Sum1/2
  Vref/1 -> Sum1/1
  Vs/1 -> Sum1/3
  Sum1/1 -> AVR SEXS/1(dV)
  AVR SEXS/1(Ef) -> Ef/1

== system IEEE_39_IBR_Simplified/A2/G1/Controllers/Governor Simplified ==
  dw : Inport
  Pref : Inport  Port=2
  Gain : Gain  Gain=Kg(1)/Rg(1)
  Saturation : Saturate  UpperLimit=Vmax  LowerLimit=Vmin
  Sum1 : Sum  Inputs=|+-
  Transfer Fcn : TransferFcn  Numerator=[Fg(1)*Tg(1) 1]  Denominator=[Tg(1) 1]
  Pm : Outport  VectorParamsAs1DForOutWhenUnconnected=off
  wires:
  Transfer Fcn/1 -> Gain/1
  dw/1 -> Transfer Fcn/1
  Pref/1 -> Sum1/1
  Sum1/1 -> Saturation/1
  Gain/1 -> Sum1/2
  Saturation/1 -> Pm/1

== system IEEE_39_IBR_Simplified/A2/G1/Controllers/Governor IEEE TGOV1 ==
  dw : Inport
  Pref : Inport  Port=2
  Gain : Gain  Gain=1/R
  Gain1 : Gain  Gain=Dt
  Saturation : Saturate  UpperLimit=Vmax  LowerLimit=Vmin
  Scope : Scope  NumInputPorts=3
  Scope1 : Scope
  Sum : Sum  Inputs=|+-
  Sum1 : Sum  Inputs=|+-
  Transfer Fcn : TransferFcn  Denominator=[T1 1]
  Transfer Fcn1 : TransferFcn  Numerator=[T2 1]  Denominator=[T3 1]
  Transfer Fcn2 : TransferFcn  Numerator=[1 1]  Denominator=[10 1]
  Pm : Outport  VectorParamsAs1DForOutWhenUnconnected=off
  wires:
  Transfer Fcn/1 -> Scope1/1, Saturation/1
  Sum1/1 -> Scope/2, Transfer Fcn/1
  Gain1/1 -> Sum/2
  Saturation/1 -> Transfer Fcn1/1
  Sum/1 -> Pm/1
  dw/1 -> Transfer Fcn2/1
  Transfer Fcn1/1 -> Scope/3, Sum/1
  Gain/1 -> Sum1/2
  Pref/1 -> Scope/1, Sum1/1
  Transfer Fcn2/1 -> Gain1/1, Gain/1

== system IEEE_39_IBR_Simplified/A2/G1/Controllers/PSS IEEE PSS1A ==
  dP : Inport
  Gain : Gain  Gain=Ks
  Transfer Fcn : TransferFcn  Numerator=[Ts1 1]  Denominator=[Ts2 1]
  Transfer Fcn1 : TransferFcn  Numerator=[Ts5 0]  Denominator=[Ts5 1]
  Transfer Fcn2 : TransferFcn  Numerator=[Ts3 1]  Denominator=[Ts4 1]
  Vs : Outport  VectorParamsAs1DForOutWhenUnconnected=off
  wires:
  Transfer Fcn/1 -> Transfer Fcn2/1
  Gain/1 -> Transfer Fcn1/1
  dP/1 -> Transfer Fcn/1
  Transfer Fcn2/1 -> Gain/1
  Transfer Fcn1/1 -> Vs/1

== system IEEE_39_IBR_Simplified/A2/G2/Controllers/AVR IEEE SEXS\ST1A ==
  Vc : Inport
  Vs : Inport  Port=2
  Vref : Inport  Port=3
  AVR IEEE ST1a : Subsystem  Commented=on
  AVR SEXS : Subsystem
  Sum1 : Sum  Inputs=+-+
  Ef : Outport  VectorParamsAs1DForOutWhenUnconnected=off
  wires:
  Vc/1 -> Sum1/2
  Vref/1 -> Sum1/1
  Vs/1 -> Sum1/3
  Sum1/1 -> AVR SEXS/1(dV)
  AVR SEXS/1(Ef) -> Ef/1

== system IEEE_39_IBR_Simplified/A2/G2/Controllers/Governor Simplified ==
  dw : Inport
  Pref : Inport  Port=2
  Gain : Gain  Gain=Kg(1)/Rg(1)
  Saturation : Saturate  UpperLimit=Vmax  LowerLimit=Vmin
  Sum1 : Sum  Inputs=|+-
  Transfer Fcn : TransferFcn  Numerator=[Fg(1)*Tg(1) 1]  Denominator=[Tg(1) 1]
  Pm : Outport  VectorParamsAs1DForOutWhenUnconnected=off
  wires:
  Transfer Fcn/1 -> Gain/1
  dw/1 -> Transfer Fcn/1
  Pref/1 -> Sum1/1
  Sum1/1 -> Saturation/1
  Gain/1 -> Sum1/2
  Saturation/1 -> Pm/1

== system IEEE_39_IBR_Simplified/A2/G2/Controllers/Governor IEEE TGOV1 ==
  dw : Inport
  Pref : Inport  Port=2
  Gain : Gain  Gain=1/R
  Gain1 : Gain  Gain=Dt
  Saturation : Saturate  UpperLimit=Vmax  LowerLimit=Vmin
  Scope : Scope  NumInputPorts=3
  Sum : Sum  Inputs=|+-
  Sum1 : Sum  Inputs=|+-
  Transfer Fcn : TransferFcn  Denominator=[T1 1]
  Transfer Fcn1 : TransferFcn  Numerator=[T2 1]  Denominator=[T3 1]
  Transfer Fcn2 : TransferFcn  Numerator=[1 1]  Denominator=[10 1]
  Pm : Outport  VectorParamsAs1DForOutWhenUnconnected=off
  wires:
  Transfer Fcn/1 -> Saturation/1
  Sum1/1 -> Scope/2, Transfer Fcn/1
  Gain1/1 -> Sum/2
  Saturation/1 -> Transfer Fcn1/1
  Sum/1 -> Pm/1
  dw/1 -> Transfer Fcn2/1
  Transfer Fcn1/1 -> Scope/3, Sum/1
  Gain/1 -> Sum1/2
  Pref/1 -> Scope/1, Sum1/1
  Transfer Fcn2/1 -> Gain1/1, Gain/1

== system IEEE_39_IBR_Simplified/A2/G2/Controllers/PSS IEEE PSS1A ==
  dP : Inport
  Gain : Gain  Gain=Ks
  Transfer Fcn : TransferFcn  Numerator=[Ts1 1]  Denominator=[Ts2 1]
  Transfer Fcn1 : TransferFcn  Numerator=[Ts5 0]  Denominator=[Ts5 1]
  Transfer Fcn2 : TransferFcn  Numerator=[Ts3 1]  Denominator=[Ts4 1]
  Vs : Outport  VectorParamsAs1DForOutWhenUnconnected=off
  wires:
  Transfer Fcn/1 -> Transfer Fcn2/1
  Gain/1 -> Transfer Fcn1/1
  dP/1 -> Transfer Fcn/1
  Transfer Fcn2/1 -> Gain/1
  Transfer Fcn1/1 -> Vs/1

== system IEEE_39_IBR_Simplified/A2/G3/Controllers/AVR IEEE SEXS\ST1A ==
  Vc : Inport
  Vs : Inport  Port=2
  Vref : Inport  Port=3
  AVR IEEE ST1a : Subsystem  Commented=on
  AVR SEXS : Subsystem
  Scope : Scope  NumInputPorts=2
  Sum1 : Sum  Inputs=+-+
  Ef : Outport  VectorParamsAs1DForOutWhenUnconnected=off
  wires:
  Vc/1 -> Sum1/2
  Vs/1 -> Sum1/3
  Sum1/1 -> Scope/1, AVR SEXS/1(dV)
  AVR SEXS/1(Ef) -> Ef/1, Scope/2
  Vref/1 -> Sum1/1

== system IEEE_39_IBR_Simplified/A2/G3/Controllers/Governor Simplified ==
  dw : Inport
  Pref : Inport  Port=2
  Gain : Gain  Gain=Kg(1)/Rg(1)
  Saturation : Saturate  UpperLimit=Vmax  LowerLimit=Vmin
  Sum1 : Sum  Inputs=|+-
  Transfer Fcn : TransferFcn  Numerator=[Fg(1)*Tg(1) 1]  Denominator=[Tg(1) 1]
  Pm : Outport  VectorParamsAs1DForOutWhenUnconnected=off
  wires:
  Transfer Fcn/1 -> Gain/1
  dw/1 -> Transfer Fcn/1
  Pref/1 -> Sum1/1
  Sum1/1 -> Saturation/1
  Gain/1 -> Sum1/2
  Saturation/1 -> Pm/1

== system IEEE_39_IBR_Simplified/A2/G3/Controllers/Governor IEEE TGOV1 ==
  dw : Inport
  Pref : Inport  Port=2
  Gain : Gain  Gain=1/R
  Gain1 : Gain  Gain=Dt
  Saturation : Saturate  UpperLimit=Vmax  LowerLimit=Vmin
  Scope : Scope  NumInputPorts=3
  Sum : Sum  Inputs=|+-
  Sum1 : Sum  Inputs=|+-
  Transfer Fcn : TransferFcn  Denominator=[T1 1]
  Transfer Fcn1 : TransferFcn  Numerator=[T2 1]  Denominator=[T3 1]
  Transfer Fcn2 : TransferFcn  Numerator=[1 1]  Denominator=[10 1]
  Pm : Outport  VectorParamsAs1DForOutWhenUnconnected=off
  wires:
  Sum1/1 -> Transfer Fcn/1, Scope/2
  Gain1/1 -> Sum/2
  Sum/1 -> Pm/1
  Saturation/1 -> Transfer Fcn1/1
  Gain/1 -> Sum1/2
  Pref/1 -> Scope/1, Sum1/1
  dw/1 -> Transfer Fcn2/1
  Transfer Fcn2/1 -> Gain1/1, Gain/1
  Transfer Fcn/1 -> Saturation/1
  Transfer Fcn1/1 -> Scope/3, Sum/1

== system IEEE_39_IBR_Simplified/A2/G3/Controllers/PSS IEEE PSS1A ==
  dP : Inport
  Gain : Gain  Gain=Ks
  Transfer Fcn : TransferFcn  Numerator=[Ts1 1]  Denominator=[Ts2 1]
  Transfer Fcn1 : TransferFcn  Numerator=[Ts5 0]  Denominator=[Ts5 1]
  Transfer Fcn2 : TransferFcn  Numerator=[Ts3 1]  Denominator=[Ts4 1]
  Vs : Outport  VectorParamsAs1DForOutWhenUnconnected=off
  wires:
  Transfer Fcn/1 -> Transfer Fcn2/1
  Gain/1 -> Transfer Fcn1/1
  dP/1 -> Transfer Fcn/1
  Transfer Fcn2/1 -> Gain/1
  Transfer Fcn1/1 -> Vs/1

== system IEEE_39_IBR_Simplified/A3/G4/Controllers/AVR IEEE SEXS\ST1A ==
  Vc : Inport
  Vs : Inport  Port=2
  Vref : Inport  Port=3
  AVR IEEE ST1a : Subsystem  Commented=on
  AVR SEXS : Subsystem
  Sum1 : Sum  Inputs=+-+
  Ef : Outport  VectorParamsAs1DForOutWhenUnconnected=off
  wires:
  Vc/1 -> Sum1/2
  Vref/1 -> Sum1/1
  Vs/1 -> Sum1/3
  Sum1/1 -> AVR SEXS/1(dV)
  AVR SEXS/1(Ef) -> Ef/1

== system IEEE_39_IBR_Simplified/A3/G4/Controllers/Governor Simplified ==
  dw : Inport
  Pref : Inport  Port=2
  Gain : Gain  Gain=Kg(1)/Rg(1)
  Saturation : Saturate  UpperLimit=Vmax  LowerLimit=Vmin
  Sum1 : Sum  Inputs=|+-
  Transfer Fcn : TransferFcn  Numerator=[Fg(1)*Tg(1) 1]  Denominator=[Tg(1) 1]
  Pm : Outport  VectorParamsAs1DForOutWhenUnconnected=off
  wires:
  Transfer Fcn/1 -> Gain/1
  dw/1 -> Transfer Fcn/1
  Pref/1 -> Sum1/1
  Sum1/1 -> Saturation/1
  Gain/1 -> Sum1/2
  Saturation/1 -> Pm/1

== system IEEE_39_IBR_Simplified/A3/G4/Controllers/Governor IEEE TGOV1 ==
  dw : Inport
  Pref : Inport  Port=2
  Gain : Gain  Gain=1/R
  Gain1 : Gain  Gain=Dt
  Saturation : Saturate  UpperLimit=Vmax  LowerLimit=Vmin
  Scope : Scope  NumInputPorts=3
  Sum : Sum  Inputs=|+-
  Sum1 : Sum  Inputs=|+-
  Transfer Fcn : TransferFcn  Denominator=[T1 1]
  Transfer Fcn1 : TransferFcn  Numerator=[T2 1]  Denominator=[T3 1]
  Transfer Fcn2 : TransferFcn  Numerator=[1 1]  Denominator=[10 1]
  Pm : Outport  VectorParamsAs1DForOutWhenUnconnected=off
  wires:
  Transfer Fcn/1 -> Saturation/1
  Sum1/1 -> Scope/2, Transfer Fcn/1
  Gain1/1 -> Sum/2
  Saturation/1 -> Transfer Fcn1/1
  Sum/1 -> Pm/1
  dw/1 -> Transfer Fcn2/1
  Transfer Fcn1/1 -> Scope/3, Sum/1
  Gain/1 -> Sum1/2
  Pref/1 -> Scope/1, Sum1/1
  Transfer Fcn2/1 -> Gain1/1, Gain/1

== system IEEE_39_IBR_Simplified/A3/G4/Controllers/PSS IEEE PSS1A ==
  dP : Inport
  Gain : Gain  Gain=Ks
  Transfer Fcn : TransferFcn  Numerator=[Ts1 1]  Denominator=[Ts2 1]
  Transfer Fcn1 : TransferFcn  Numerator=[Ts5 0]  Denominator=[Ts5 1]
  Transfer Fcn2 : TransferFcn  Numerator=[Ts3 1]  Denominator=[Ts4 1]
  Vs : Outport  VectorParamsAs1DForOutWhenUnconnected=off
  wires:
  Transfer Fcn/1 -> Transfer Fcn2/1
  Gain/1 -> Transfer Fcn1/1
  dP/1 -> Transfer Fcn/1
  Transfer Fcn2/1 -> Gain/1
  Transfer Fcn1/1 -> Vs/1

== system IEEE_39_IBR_Simplified/A3/G5/Controllers/AVR IEEE SEXS\ST1A ==
  Vc : Inport
  Vs : Inport  Port=2
  Vref : Inport  Port=3
  AVR IEEE ST1a : Subsystem  Commented=on
  AVR SEXS : Subsystem
  Sum1 : Sum  Inputs=+-+
  Ef : Outport  VectorParamsAs1DForOutWhenUnconnected=off
  wires:
  Vc/1 -> Sum1/2
  Vref/1 -> Sum1/1
  Vs/1 -> Sum1/3
  Sum1/1 -> AVR SEXS/1(dV)
  AVR SEXS/1(Ef) -> Ef/1

== system IEEE_39_IBR_Simplified/A3/G5/Controllers/Governor Simplified ==
  dw : Inport
  Pref : Inport  Port=2
  Gain : Gain  Gain=Kg(1)/Rg(1)
  Saturation : Saturate  UpperLimit=Vmax  LowerLimit=Vmin
  Sum1 : Sum  Inputs=|+-
  Transfer Fcn : TransferFcn  Numerator=[Fg(1)*Tg(1) 1]  Denominator=[Tg(1) 1]
  Pm : Outport  VectorParamsAs1DForOutWhenUnconnected=off
  wires:
  Transfer Fcn/1 -> Gain/1
  dw/1 -> Transfer Fcn/1
  Pref/1 -> Sum1/1
  Sum1/1 -> Saturation/1
  Gain/1 -> Sum1/2
  Saturation/1 -> Pm/1

== system IEEE_39_IBR_Simplified/A3/G5/Controllers/Governor IEEE TGOV1 ==
  dw : Inport
  Pref : Inport  Port=2
  Gain : Gain  Gain=1/R
  Gain1 : Gain  Gain=Dt
  Saturation : Saturate  UpperLimit=Vmax  LowerLimit=Vmin
  Scope : Scope  NumInputPorts=3
  Sum : Sum  Inputs=|+-
  Sum1 : Sum  Inputs=|+-
  Transfer Fcn : TransferFcn  Denominator=[T1 1]
  Transfer Fcn1 : TransferFcn  Numerator=[T2 1]  Denominator=[T3 1]
  Transfer Fcn2 : TransferFcn  Numerator=[1 1]  Denominator=[10 1]
  Pm : Outport  VectorParamsAs1DForOutWhenUnconnected=off
  wires:
  Transfer Fcn/1 -> Saturation/1
  Sum1/1 -> Scope/2, Transfer Fcn/1
  Gain1/1 -> Sum/2
  Saturation/1 -> Transfer Fcn1/1
  Sum/1 -> Pm/1
  dw/1 -> Transfer Fcn2/1
  Transfer Fcn1/1 -> Scope/3, Sum/1
  Gain/1 -> Sum1/2
  Pref/1 -> Scope/1, Sum1/1
  Transfer Fcn2/1 -> Gain1/1, Gain/1

== system IEEE_39_IBR_Simplified/A3/G5/Controllers/PSS IEEE PSS1A ==
  dP : Inport
  Gain : Gain  Gain=Ks
  Transfer Fcn : TransferFcn  Numerator=[Ts1 1]  Denominator=[Ts2 1]
  Transfer Fcn1 : TransferFcn  Numerator=[Ts5 0]  Denominator=[Ts5 1]
  Transfer Fcn2 : TransferFcn  Numerator=[Ts3 1]  Denominator=[Ts4 1]
  Vs : Outport  VectorParamsAs1DForOutWhenUnconnected=off
  wires:
  Transfer Fcn/1 -> Transfer Fcn2/1
  Gain/1 -> Transfer Fcn1/1
  dP/1 -> Transfer Fcn/1
  Transfer Fcn2/1 -> Gain/1
  Transfer Fcn1/1 -> Vs/1

== system IEEE_39_IBR_Simplified/A3/G6/Controllers/AVR IEEE SEXS\ST1A ==
  Vc : Inport
  Vs : Inport  Port=2
  Vref : Inport  Port=3
  AVR IEEE ST1a : Subsystem  Commented=on
  AVR SEXS : Subsystem
  Sum1 : Sum  Inputs=+-+
  Ef : Outport  VectorParamsAs1DForOutWhenUnconnected=off
  wires:
  Vc/1 -> Sum1/2
  Vref/1 -> Sum1/1
  Vs/1 -> Sum1/3
  Sum1/1 -> AVR SEXS/1(dV)
  AVR SEXS/1(Ef) -> Ef/1

== system IEEE_39_IBR_Simplified/A3/G6/Controllers/Governor Simplified ==
  dw : Inport
  Pref : Inport  Port=2
  Gain : Gain  Gain=Kg(1)/Rg(1)
  Saturation : Saturate  UpperLimit=Vmax  LowerLimit=Vmin
  Sum1 : Sum  Inputs=|+-
  Transfer Fcn : TransferFcn  Numerator=[Fg(1)*Tg(1) 1]  Denominator=[Tg(1) 1]
  Pm : Outport  VectorParamsAs1DForOutWhenUnconnected=off
  wires:
  Transfer Fcn/1 -> Gain/1
  dw/1 -> Transfer Fcn/1
  Pref/1 -> Sum1/1
  Sum1/1 -> Saturation/1
  Gain/1 -> Sum1/2
  Saturation/1 -> Pm/1
